simulink model "ctrl_30khz"  (R2017a)
settings: Solver=FixedStepDiscrete  StartTime=0.0  StopTime=10.0  RelTol=1e-3  EnableMultiTasking=on
libraries: ctrl_lib x3
settings Model: Creator=uids8840  LastModifiedBy=root
settings SolverCC: AutoInsertRateTranBlk=on
settings DataIOCC: SaveOutput=off  SignalLogging=off  DSMLogging=off  SaveTime=off
settings OptimizationCC: DefaultParameterBehavior=Inlined  UseFloatMulNetSlope=on  DefaultUnderspecifiedDataType=single  InlineInvariantSignals=on  PassReuseOutputArgsAs=Individual arguments  ZeroExternalMemoryAtStartup=off  ZeroInternalMemoryAtStartup=off  NoFixptDivByZeroProtection=on  EfficientFloat2IntCast=on  LifeSpan=1
settings DebuggingCC: ParameterTunabilityLossMsg=error
settings HardwareCC: ProdBitPerPointer=32  ProdBitPerSizeT=32  ProdBitPerPtrDiffT=32  ProdLargestAtomicInteger=Long  ProdLargestAtomicFloat=Double  ProdWordSize=32  ProdLongLongMode=on  ProdHWDeviceType=ARM Compatible->ARM Cortex
settings ModelReferenceCC: ModelReferenceNumInstancesAllowed=Single
settings SFSimCC: MATLABDynamicMemAlloc=off
settings RTWCC: SystemTargetFile=ert.tlc  GenCodeOnly=on  PackageGeneratedCodeAndArtifacts=on  PackageName=mtrctl  TemplateMakefile=ert_default_tmf  Description=Embedded Coder  GenerateReport=on  IncludeHyperlinkInReport=on  LaunchReport=on  GenerateTraceInfo=on  GenerateTraceReport=on  GenerateTraceReportSl=on  GenerateTraceReportSf=on  GenerateTraceReportEml=on  GenerateCodeMetricsReport=on
settings CodeAppCC: ForceParamTrailComments=on  IgnoreCustomStorageClasses=off  OperatorAnnotations=on  SimulinkDataObjDesc=on  SFDataObjDesc=on  CustomSymbolStrGlobalVar=rt$N$M  CustomSymbolStrType=$N$M  CustomSymbolStrFcn=$N$M$F  CustomSymbolStrMacro=$N$M  InsertBlockDesc=on
settings ERTTargetCC: TargetLangStandard=C99 (ISO)  GenerateFullHeader=off  IncludeMdlTerminateFcn=off  CombineSignalStateStructs=on  SuppressErrorStatus=on  ERTCustomFileBanners=off  SupportAbsoluteTime=off  SupportNonFinite=off  SupportComplex=off  InlinedParameterPlacement=NonHierarchical  ERTCustomFileTemplate=example_file_process.tlc  GlobalDataDefinition=InSourceFile  GlobalDataReference=InSourceFile  ERTFilePackagingFormat=CompactWithDataFile

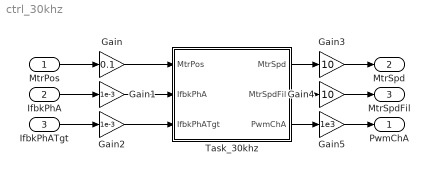
== system ctrl_30khz ==
  MtrPos : Inport
  IfbkPhA : Inport  Port=2
  IfbkPhATgt : Inport  Port=3
  Gain : Gain  Gain=0.1
  Gain1 : Gain  Gain=1e-3
  Gain2 : Gain  Gain=1e-3
  Gain3 : Gain  Gain=10
  Gain4 : Gain  Gain=10
  Gain5 : Gain  Gain=1e3
  Task_30khz : Subsystem  SystemSampleTime=1/30e3
      settings: RTWFcnNameOpts=Use subsystem name  RTWFileNameOpts=Use subsystem name
  PwmChA : Outport
  MtrSpd : Outport  Port=2
  MtrSpdFil : Outport  Port=3
  wires:
  MtrPos/1 -> Gain/1
  Task_30khz/3(PwmChA) -> Gain5/1
  IfbkPhA/1 -> Gain1/1
  Task_30khz/1(MtrSpd) -> Gain3/1
  Task_30khz/2(MtrSpdFil) -> Gain4/1
  IfbkPhATgt/1 -> Gain2/1
  Gain/1 -> Task_30khz/1(MtrPos)
  Gain1/1 -> Task_30khz/2(IfbkPhA)
  Gain2/1 -> Task_30khz/3(IfbkPhATgt)
  Gain3/1 -> MtrSpd/1
  Gain4/1 -> MtrSpdFil/1
  Gain5/1 -> PwmChA/1

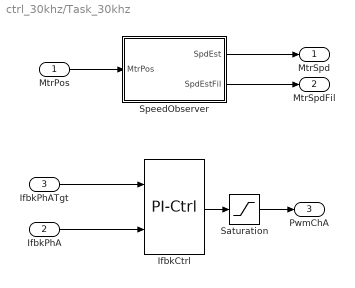
== system ctrl_30khz/Task_30khz ==
  MtrPos : Inport
  IfbkPhA : Inport  Port=2
  IfbkPhATgt : Inport  Port=3
  IfbkCtrl : ctrl_lib/PI-Ctrl  ts=1/30e3  PI_Kp=Ifbk_PI_Kp  PI_Ki=Ifbk_PI_Ki
  Saturation : Saturate  UpperLimit=12  LowerLimit=-12
  SpeedObserver : Subsystem  RTWFcnName=SpdEst  RTWFileName=spdest
      settings: RTWFcnNameOpts=Use subsystem name  RTWFileNameOpts=Use subsystem name
  MtrSpd : Outport
  MtrSpdFil : Outport  Port=2
  PwmChA : Outport  Port=3
  wires:
  SpeedObserver/2(SpdEstFil) -> MtrSpdFil/1
  SpeedObserver/1(SpdEst) -> MtrSpd/1
  IfbkPhA/1 -> IfbkCtrl/2
  MtrPos/1 -> SpeedObserver/1(MtrPos)
  IfbkPhATgt/1 -> IfbkCtrl/1
  IfbkCtrl/1 -> Saturation/1
  Saturation/1 -> PwmChA/1

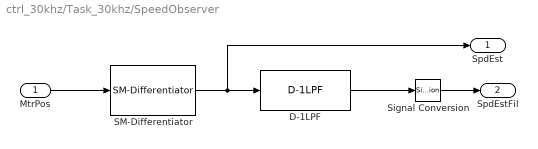
== system ctrl_30khz/Task_30khz/SpeedObserver ==
  MtrPos : Inport
  D-1LPF : ctrl_lib/D-1LPF  k_filt=Spd_SMDiff_Filt_K
  SM-Differentiator : ctrl_lib/SM-Differentiator  sm_ki=Pos_SMDiff_Ki  sm_kp=Pos_SMDiff_Kp  ts=1/30e3
  Signal Conversion : SignalConversion  OverrideOpt=off
  SpdEst : Outport
  SpdEstFil : Outport  Port=2
  wires:
  SM-Differentiator/1 -> SpdEst/1, D-1LPF/1
  D-1LPF/1 -> Signal Conversion/1
  MtrPos/1 -> SM-Differentiator/1
  Signal Conversion/1 -> SpdEstFil/1
